simulink subsystem "LED_Strip_Avg"  (R2023b)
settings: Solver=VariableStepAuto  StartTime=0.0  StopTime=10.0  RelTol=1e-3
libraries: fl_lib x2
settings Model: Creator=vlenzi  LastModifiedBy=vlenzi

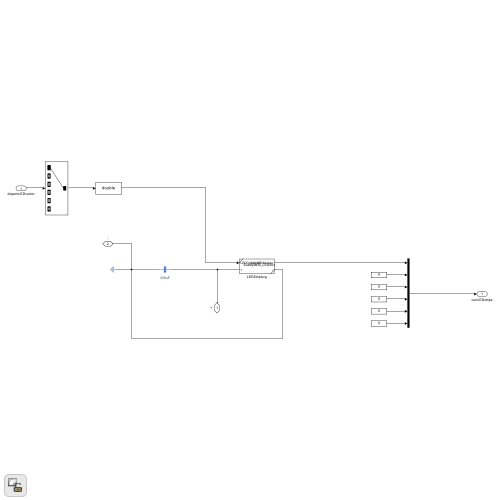
[thumbnail: Simulink's stored preview of the top-level diagram]
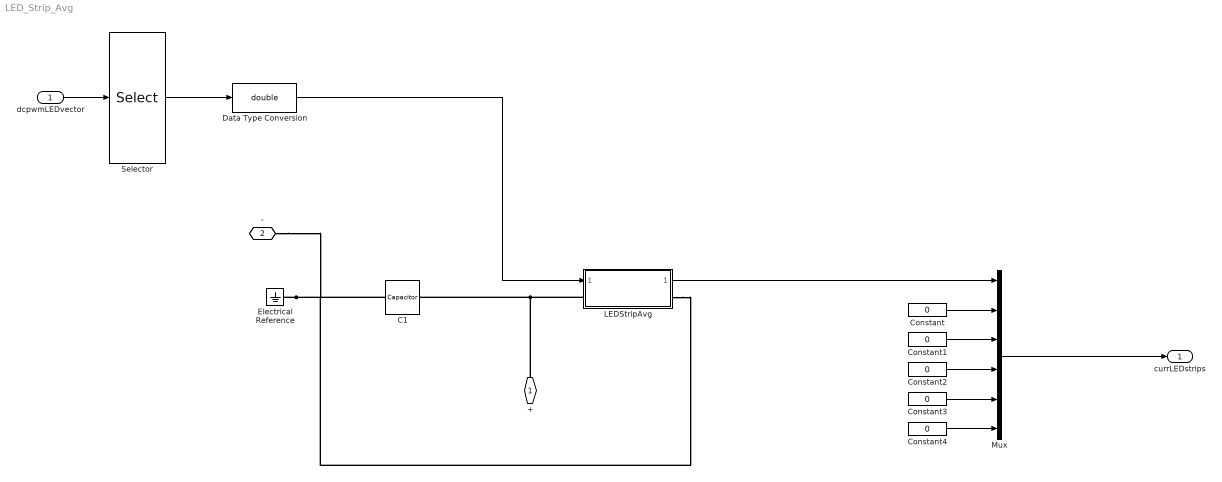
== system LED_Strip_Avg ==
  dcpwmLEDvector : Inport
  C1 : fl_lib/Electrical/Electrical Elements/Capacitor  c=330 uF  r=1e-6 Ohm  g=0 1/Ohm  i_specify=off  i_priority=None  i=0 A  i_nominal_specify=off  i_nominal_unit=A  i_nominal_value=1  v_specify=off  v_priority=None  v=0 V  v_nominal_specify=off  v_nominal_unit=V  v_nominal_value=1  vc_specify=off  vc_priority=High  vc=0 V  vc_nominal_specify=off  vc_nominal_unit=V  vc_nominal_value=1
      settings: AttributesFormatString=%<c>%<c_unit>
  Constant{,1..4} (5 alike) : Constant  Value=0
  Data Type Conversion : DataTypeConversion  OutDataTypeStr=double  SaturateOnIntegerOverflow=off  RndMeth=Floor
  Electrical Reference : fl_lib/Electrical/Electrical Elements/Electrical Reference
  LEDStripAvg : Subsystem  ReferencedSubsystem=Subsystem_LEDStripAvg
  Mux : Mux  Inputs=6
  Selector : Selector  InputPortWidth=6  IndexOptions=Index vector (dialog)  Indices=[1]  OutputSizes=1
  + : PMIOPort  Side=Left
  - : PMIOPort  Port=2  Side=Right
  currLEDstrips : Outport  Unit=mA  VectorParamsAs1DForOutWhenUnconnected=off
  wires:
  Data Type Conversion/1 -> LEDStripAvg/1
  Mux/1 -> currLEDstrips/1
  Constant4/1 -> Mux/6
  Constant3/1 -> Mux/5
  Constant2/1 -> Mux/4
  Constant1/1 -> Mux/3
  Constant/1 -> Mux/2
  Selector/1 -> Data Type Conversion/1
  dcpwmLEDvector/1 -> Selector/1
  LEDStripAvg/1 -> Mux/1
  connections:
  Electrical Reference/LConn1 -- -/RConn1 -- C1/RConn1 -- LEDStripAvg/RConn1
  +/RConn1 -- LEDStripAvg/LConn1 -- C1/LConn1
